simulink library "monroe_library"  (R2012b)
settings: Solver=ode45  StartTime=0.0  StopTime=10.0  RelTol=1e-3
values from neighbouring files (symbols this model uses):
  input_bit_width = ', num2str(input_bit_width))    [fft_direct_draw.m]
undefined symbols (not defined in the file or in its folder): gcbh, xlBlockLoadCallback
libraries: xbsIndex_r4 x1880, monroe_library x159, casper_library x13, xps_library x1
(part 11 of 43)

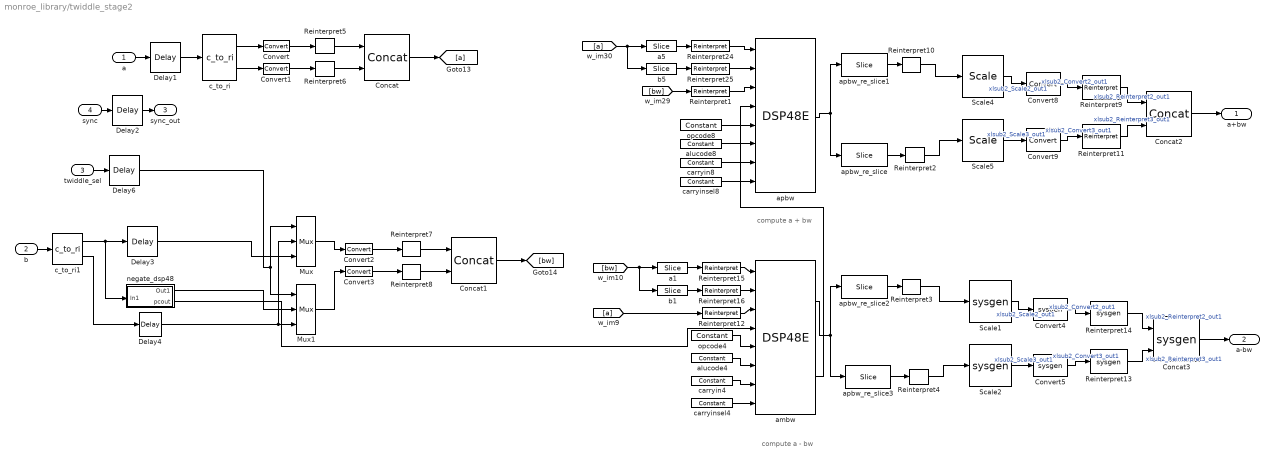
== system monroe_library/twiddle_stage2 ==
  note: compute a + bw
  note: compute a - bw
  a : Inport
  b : Inport  Port=2
  twiddle_sel : Inport  Port=3
  sync : Inport  Port=4
  Concat : xbsIndex_r4/Concat  num_inputs=2  dbl_ovrd=off  block_type=concat
      settings: block_version=11.3
  Concat1 : xbsIndex_r4/Concat  num_inputs=2  dbl_ovrd=off  block_type=concat
      settings: block_version=11.3
  Concat2 : xbsIndex_r4/Concat  num_inputs=2  dbl_ovrd=off  block_type=concat
  Concat3 : S-Function  LoadFcn=xlBlockLoadCallback(gcbh);  FunctionName=sysgen  Parameters=ptable_  EnableBusSupport=off  mask(Xilinx Bus Concatenator Block){infoedit=Concatenates two or more inputs.  Output will be cast to an unsigned value with the binary point at zero., num_inputs=2, dbl_ovrd_sgadvanced=, dbl_ovrd=off, has_advanced_control=0, sggui_pos=-1,-1,-1,-1, block_type=concat, block_version=, sg_icon_stat=60,60,2,1,white,blue,0,16398980,right,,[ ],[ ], sg_mask_display=|, sg_list_contents=, sg_blockgui_xml=}
      mask sg_mask_display=|
      | fprintf('','COMMENT: begin icon graphics');
      | patch([0 60 60 0 0 ],[0 0 60 60 0 ],[0.77 0.82 0.91 ]);
      | plot([0 60 60 0 0 ],[0 0 60 60 0 ]);
      | patch([12.2 23.76 31.76 39.76 47.76 31.76 20.2 12.2 ],[38.88 38.88 46.88 38.88 46.88 46.88 46.88 38.88 ],[1 1 1 ]);
      | patch([20.2 31.76 23.76 12.2 20.2 ],[30.88 30.88 38.88 38.88 30.88 ],[0.931 0.946 0.973 ]);
      | patch([12.2 23.76 31.76 20.2 12.2 ],[22.88 22.88 30.88 30.88 22.88 ],[1 1 1 ]);
      | patch([20.2 47.76 39.76 31.76 23.76 12.2 20.2 ],[14.88 14.88 22.88 14.88 22.88 22.88 14.88 ],[0.931 0.946 0.973 ]);
      | fprintf('','COMMENT: end icon graphics');
      | fprintf('','COMMENT: begin icon text');
      | color('black');port_label('input',1,'hi');
      | color('black');port_label('input',2,'lo');
      |
      | color('black');disp('\fontsize{20}\}','texmode','on');
      | fprintf('','COMMENT: end icon text');
      mask prompts: infoedit ""; num_inputs "Number of inputs"; dbl_ovrd_sgadvanced ""; dbl_ovrd "Override with doubles"; has_advanced_control ""; sggui_pos ""; block_type ""; block_version ""; sg_icon_stat ""; sg_mask_display ""; sg_list_contents ""; sg_blockgui_xml ""
      mask help: Concatenates two or more inputs. Output will be cast to an unsigned value with the binary point at zero.
      mask init: same as monroe_library/double_delay_bram_external_counter/Concat1
      settings: CopyFcn=xlBlockMoveCallback(gcbh);  DeleteFcn=xlDestroyGui(gcbh);  ModelCloseFcn=xlDestroyGui(gcbh);  PreSaveFcn=xlBlockPreSaveCallback(gcbh);  PostSaveFcn=xlBlockPostSaveCallback(gcbh);  DestroyFcn=xlDestroyGui(gcbh);  OpenFcn=xlOpenGui(gcbh, 'concat_gui.xml', @xlmagicenablement, -1)  CloseFcn=xlDestroyGui(gcbh);  MoveFcn=xlBlockMoveCallback(gcbh);
      mask Help: eval('');xlDoc('-book','sysgen','-topic','Concat');
      mask Display:
      | fprintf('','COMMENT: begin icon graphics');
      | patch([0 60 60 0 0 ],[0 0 60 60 0 ],[0.77 0.82 0.91 ]);
      | plot([0 60 60 0 0 ],[0 0 60 60 0 ]);
      | patch([12.2 23.76 31.76 39.76 47.76 31.76 20.2 12.2 ],[38.88 38.88 46.88 38.88 46.88 46.88 46.88 38.88 ],[1 1 1 ]);
      | patch([20.2 31.76 23.76 12.2 20.2 ],[30.88 30.88 38.88 38.88 30.88 ],[0.931 0.946 0.973 ]);
      | patch([12.2 23.76 31.76 20.2 12.2 ],[22.88 22.88 30.88 30.88 22.88 ],[1 1 1 ]);
      | patch([20.2 47.76 39.76 31.76 23.76 12.2 20.2 ],[14.88 14.88 22.88 14.88 22.88 22.88 14.88 ],[0.931 0.946 0.973 ]);
      | fprintf('','COMMENT: end icon graphics');
      | fprintf('','COMMENT: begin icon text');
      | color('black');port_label('input',1,'hi');
      | color('black');port_label('input',2,'lo');
      | 
      | color('black');disp('\fontsize{20}\}','texmode','on');
      | fprintf('','COMMENT: end icon text');
  Convert{,1..3} (4 alike) : xbsIndex_r4/Convert  arith_type="Signed  (2's comp)"  n_bits=24  bin_pt=input_bit_width-1  quantization=Truncate  overflow=Wrap  en=off  latency=0  dbl_ovrd=off  pipeline=off  block_type=convert
      settings: block_version=11.4
  Convert4 : S-Function  LoadFcn=xlBlockLoadCallback(gcbh);  FunctionName=sysgen  Parameters=ptable_  EnableBusSupport=off  mask(Xilinx Type Converter Block){infoedit=Hardware notes: rounding and saturating require hardware resources; truncating and wrapping do not., arith_type_sgadvanced=, arith_type=Signed  (2's comp), n_bits=out_n_bits, bin_pt=out_n_bits-1, quantization_sgadvanced=, quantization=Truncate, overflow_sgadvanced=, overflow=Wrap, en_sgadvanced=, en=off, latency=0, dbl_ovrd_sgadvanced=, dbl_ovrd=off, pipeline_sgadvanced=, pipeline=off, xl_use_area_sgadvanced=, xl_use_area=off, xl_area=[0,0,0,0,0,0,0], has_advanced_control=0, sggui_pos=-1,-1,-1,-1, block_type=convert, block_version=, sg_icon_stat=45,30,1,1,white,blue,0,edca21da,right,,[ ],[ ], sg_mask_display=|, sg_list_contents=, sg_blockgui_xml=}
      mask sg_mask_display=|
      | fprintf('','COMMENT: begin icon graphics');
      | patch([0 45 45 0 0 ],[0 0 30 30 0 ],[0.77 0.82 0.91 ]);
      | plot([0 45 45 0 0 ],[0 0 30 30 0 ]);
      | patch([13.1 18.88 22.88 26.88 30.88 22.88 17.1 13.1 ],[19.44 19.44 23.44 19.44 23.44 23.44 23.44 19.44 ],[1 1 1 ]);
      | patch([17.1 22.88 18.88 13.1 17.1 ],[15.44 15.44 19.44 19.44 15.44 ],[0.931 0.946 0.973 ]);
      | patch([13.1 18.88 22.88 17.1 13.1 ],[11.44 11.44 15.44 15.44 11.44 ],[1 1 1 ]);
      | patch([17.1 30.88 26.88 22.88 18.88 13.1 17.1 ],[7.44 7.44 11.44 7.44 11.44 11.44 7.44 ],[0.931 0.946 0.973 ]);
      | fprintf('','COMMENT: end icon graphics');
      | fprintf('','COMMENT: begin icon text');
      |
      | color('black');port_label('output',1,'cast');
      | fprintf('','COMMENT: end icon text');
      mask prompts: infoedit ""; arith_type_sgadvanced ""; arith_type "Type"; n_bits "Number of bits"; bin_pt "Binary point"; quantization_sgadvanced ""; overflow_sgadvanced ""; en_sgadvanced ""; en "Provide enable port"; dbl_ovrd_sgadvanced ""; dbl_ovrd "Override with doubles"; pipeline_sgadvanced ""; pipeline "Pipeline for maximum performance"; xl_use_area_sgadvanced ""; xl_use_area "Define FPGA area for resource estimation"; xl_area "FPGA area [slices, FFs, BRAMs, LUTs, IOBs, emb. mults, TBUFs]"; has_advanced_control ""; sggui_pos ""; block_type ""; block_version ""; sg_icon_stat ""; sg_mask_display ""; sg_list_contents ""; sg_blockgui_xml ""
      mask help: Hardware notes: rounding and saturating require hardware resources; truncating and wrapping do not.
      mask init: same as monroe_library/dsp48e_mult_add_pcin/Convert
      settings: CopyFcn=xlBlockMoveCallback(gcbh);  DeleteFcn=xlDestroyGui(gcbh);  ModelCloseFcn=xlDestroyGui(gcbh);  PreSaveFcn=xlBlockPreSaveCallback(gcbh);  PostSaveFcn=xlBlockPostSaveCallback(gcbh);  DestroyFcn=xlDestroyGui(gcbh);  OpenFcn=xlOpenGui(gcbh, 'convert_gui.xml', @convertenablement, -1)  CloseFcn=xlDestroyGui(gcbh);  MoveFcn=xlBlockMoveCallback(gcbh);
      mask Help: eval('');xlDoc('-book','sysgen','-topic','Convert');
      mask TypeOptions arith_type: Boolean | Signed  (2's comp) | Unsigned
      mask TypeOptions quantization: Truncate | Round  (unbiased: +/- Inf) | Round  (unbiased: Even Values)
      mask TypeOptions overflow: Wrap | Saturate | Flag as error
      mask Display:
      | fprintf('','COMMENT: begin icon graphics');
      | patch([0 45 45 0 0 ],[0 0 30 30 0 ],[0.77 0.82 0.91 ]);
      | plot([0 45 45 0 0 ],[0 0 30 30 0 ]);
      | patch([13.1 18.88 22.88 26.88 30.88 22.88 17.1 13.1 ],[19.44 19.44 23.44 19.44 23.44 23.44 23.44 19.44 ],[1 1 1 ]);
      | patch([17.1 22.88 18.88 13.1 17.1 ],[15.44 15.44 19.44 19.44 15.44 ],[0.931 0.946 0.973 ]);
      | patch([13.1 18.88 22.88 17.1 13.1 ],[11.44 11.44 15.44 15.44 11.44 ],[1 1 1 ]);
      | patch([17.1 30.88 26.88 22.88 18.88 13.1 17.1 ],[7.44 7.44 11.44 7.44 11.44 11.44 7.44 ],[0.931 0.946 0.973 ]);
      | fprintf('','COMMENT: end icon graphics');
      | fprintf('','COMMENT: begin icon text');
      | 
      | color('black');port_label('output',1,'cast');
      | fprintf('','COMMENT: end icon text');
  Convert5 : S-Function  LoadFcn=xlBlockLoadCallback(gcbh);  FunctionName=sysgen  Parameters=ptable_  EnableBusSupport=off  mask(Xilinx Type Converter Block){infoedit=Hardware notes: rounding and saturating require hardware resources; truncating and wrapping do not., arith_type_sgadvanced=, arith_type=Signed  (2's comp), n_bits=out_n_bits, bin_pt=out_n_bits-1, quantization_sgadvanced=, quantization=Truncate, overflow_sgadvanced=, overflow=Wrap, en_sgadvanced=, en=off, latency=0, dbl_ovrd_sgadvanced=, dbl_ovrd=off, pipeline_sgadvanced=, pipeline=off, xl_use_area_sgadvanced=, xl_use_area=off, xl_area=[0,0,0,0,0,0,0], has_advanced_control=0, sggui_pos=-1,-1,-1,-1, block_type=convert, block_version=, sg_icon_stat=45,30,1,1,white,blue,0,edca21da,right,,[ ],[ ], sg_mask_display=|, sg_list_contents=, sg_blockgui_xml=}
      mask sg_mask_display=|
      | fprintf('','COMMENT: begin icon graphics');
      | patch([0 45 45 0 0 ],[0 0 30 30 0 ],[0.77 0.82 0.91 ]);
      | plot([0 45 45 0 0 ],[0 0 30 30 0 ]);
      | patch([13.1 18.88 22.88 26.88 30.88 22.88 17.1 13.1 ],[19.44 19.44 23.44 19.44 23.44 23.44 23.44 19.44 ],[1 1 1 ]);
      | patch([17.1 22.88 18.88 13.1 17.1 ],[15.44 15.44 19.44 19.44 15.44 ],[0.931 0.946 0.973 ]);
      | patch([13.1 18.88 22.88 17.1 13.1 ],[11.44 11.44 15.44 15.44 11.44 ],[1 1 1 ]);
      | patch([17.1 30.88 26.88 22.88 18.88 13.1 17.1 ],[7.44 7.44 11.44 7.44 11.44 11.44 7.44 ],[0.931 0.946 0.973 ]);
      | fprintf('','COMMENT: end icon graphics');
      | fprintf('','COMMENT: begin icon text');
      |
      | color('black');port_label('output',1,'cast');
      | fprintf('','COMMENT: end icon text');
      mask prompts: infoedit ""; arith_type_sgadvanced ""; arith_type "Type"; n_bits "Number of bits"; bin_pt "Binary point"; quantization_sgadvanced ""; overflow_sgadvanced ""; en_sgadvanced ""; en "Provide enable port"; dbl_ovrd_sgadvanced ""; dbl_ovrd "Override with doubles"; pipeline_sgadvanced ""; pipeline "Pipeline for maximum performance"; xl_use_area_sgadvanced ""; xl_use_area "Define FPGA area for resource estimation"; xl_area "FPGA area [slices, FFs, BRAMs, LUTs, IOBs, emb. mults, TBUFs]"; has_advanced_control ""; sggui_pos ""; block_type ""; block_version ""; sg_icon_stat ""; sg_mask_display ""; sg_list_contents ""; sg_blockgui_xml ""
      mask help: Hardware notes: rounding and saturating require hardware resources; truncating and wrapping do not.
      mask init: same as monroe_library/dsp48e_mult_add_pcin/Convert
      settings: CopyFcn=xlBlockMoveCallback(gcbh);  DeleteFcn=xlDestroyGui(gcbh);  ModelCloseFcn=xlDestroyGui(gcbh);  PreSaveFcn=xlBlockPreSaveCallback(gcbh);  PostSaveFcn=xlBlockPostSaveCallback(gcbh);  DestroyFcn=xlDestroyGui(gcbh);  OpenFcn=xlOpenGui(gcbh, 'convert_gui.xml', @convertenablement, -1)  CloseFcn=xlDestroyGui(gcbh);  MoveFcn=xlBlockMoveCallback(gcbh);
      mask Help: eval('');xlDoc('-book','sysgen','-topic','Convert');
      mask TypeOptions arith_type: Boolean | Signed  (2's comp) | Unsigned
      mask TypeOptions quantization: Truncate | Round  (unbiased: +/- Inf) | Round  (unbiased: Even Values)
      mask TypeOptions overflow: Wrap | Saturate | Flag as error
      mask Display:
      | fprintf('','COMMENT: begin icon graphics');
      | patch([0 45 45 0 0 ],[0 0 30 30 0 ],[0.77 0.82 0.91 ]);
      | plot([0 45 45 0 0 ],[0 0 30 30 0 ]);
      | patch([13.1 18.88 22.88 26.88 30.88 22.88 17.1 13.1 ],[19.44 19.44 23.44 19.44 23.44 23.44 23.44 19.44 ],[1 1 1 ]);
      | patch([17.1 22.88 18.88 13.1 17.1 ],[15.44 15.44 19.44 19.44 15.44 ],[0.931 0.946 0.973 ]);
      | patch([13.1 18.88 22.88 17.1 13.1 ],[11.44 11.44 15.44 15.44 11.44 ],[1 1 1 ]);
      | patch([17.1 30.88 26.88 22.88 18.88 13.1 17.1 ],[7.44 7.44 11.44 7.44 11.44 11.44 7.44 ],[0.931 0.946 0.973 ]);
      | fprintf('','COMMENT: end icon graphics');
      | fprintf('','COMMENT: begin icon text');
      | 
      | color('black');port_label('output',1,'cast');
      | fprintf('','COMMENT: end icon text');
  Convert8 : xbsIndex_r4/Convert  arith_type="Signed  (2's comp)"  n_bits=out_n_bits  bin_pt=out_n_bits-1  quantization=Truncate  overflow=Wrap  en=off  latency=0  dbl_ovrd=off  pipeline=off  block_type=convert
  Convert9 : xbsIndex_r4/Convert  arith_type="Signed  (2's comp)"  n_bits=out_n_bits  bin_pt=out_n_bits-1  quantization=Truncate  overflow=Wrap  en=off  latency=0  dbl_ovrd=off  pipeline=off  block_type=convert
  Delay{1,3..4,6} (4 alike) : xbsIndex_r4/Delay  en=off  latency=3  dbl_ovrd=off  reg_retiming=off  block_type=delay
      settings: xl_area=[0, 0, 0, 0, 0, 0, 0]  block_version=9.1.01
  Delay2 : xbsIndex_r4/Delay  en=off  latency=5  dbl_ovrd=off  reg_retiming=off  block_type=delay
      settings: xl_area=[0, 0, 0, 0, 0, 0, 0]  block_version=9.1.01
  Mux : xbsIndex_r4/Mux  inputs=2  en=off  latency=0  precision=Full  arith_type="Signed  (2's comp)"  n_bits=8  bin_pt=2  quantization=Truncate  overflow=Wrap  dbl_ovrd=off  block_type=mux
      settings: xl_area=[0, 0, 0, 0, 0, 0, 0]  block_version=9.1.01
  Mux1 : xbsIndex_r4/Mux  inputs=2  en=off  latency=0  precision=Full  arith_type="Signed  (2's comp)"  n_bits=8  bin_pt=2  quantization=Truncate  overflow=Wrap  dbl_ovrd=off  block_type=mux
      settings: xl_area=[0, 0, 0, 0, 0, 0, 0]  block_version=9.1.01
  Reinterpret{1,12,15..16,24..25} (6 alike) : xbsIndex_r4/Reinterpret  force_arith_type=on  arith_type="Signed  (2's comp)"  force_bin_pt=off  bin_pt=0  block_type=reinterpret
      settings: infoedit="Changes signal type without altering the binary representation.   You can changed the signal between signed and unsigned, and relocate the binary point.<br><br>Hardware notes: In hardware this block costs nothing.<br><br>Example:  Suppose the input is 6 bits wide, signed, with 2 fractional bits, and the output is forced to unsigned with 0 fractional bits.  Then an input of -2.0 (1110.00 in binary 2's complement) becomes an output of 56 (111000 in binary)."  block_version=11.3
  Reinterpret{2..4,10} (4 alike) : xbsIndex_r4/Reinterpret  force_arith_type=on  arith_type="Signed  (2's comp)"  force_bin_pt=on  bin_pt=input_bit_width-1  block_type=reinterpret
      settings: infoedit="Changes signal type without altering the binary representation.   You can changed the signal between signed and unsigned, and relocate the binary point.<br><br>Hardware notes: In hardware this block costs nothing.<br><br>Example:  Suppose the input is 6 bits wide, signed, with 2 fractional bits, and the output is forced to unsigned with 0 fractional bits.  Then an input of -2.0 (1110.00 in binary 2's complement) becomes an output of 56 (111000 in binary)."  block_version=11.3
  Reinterpret{5..9,11} (6 alike) : xbsIndex_r4/Reinterpret  force_arith_type=on  arith_type=Unsigned  force_bin_pt=on  bin_pt=0  block_type=reinterpret
      Reinterpret11 settings: infoedit="Changes signal type without altering the binary representation.   You can changed the signal between signed and unsigned, and relocate the binary point.<br><br>Hardware notes: In hardware this block costs nothing.<br><br>Example:  Suppose the input is 6 bits wide, signed, with 2 fractional bits, and the output is forced to unsigned with 0 fractional bits.  Then an input of -2.0 (1110.00 in binary 2's complement) becomes an output of 56 (111000 in binary)."
      Reinterpret5 settings: infoedit="Changes signal type without altering the binary representation.   You can changed the signal between signed and unsigned, and relocate the binary point.<br><br>Hardware notes: In hardware this block costs nothing.<br><br>Example:  Suppose the input is 6 bits wide, signed, with 2 fractional bits, and the output is forced to unsigned with 0 fractional bits.  Then an input of -2.0 (1110.00 in binary 2's complement) becomes an output of 56 (111000 in binary)."  block_version=11.3
      Reinterpret6 settings: infoedit="Changes signal type without altering the binary representation.   You can changed the signal between signed and unsigned, and relocate the binary point.<br><br>Hardware notes: In hardware this block costs nothing.<br><br>Example:  Suppose the input is 6 bits wide, signed, with 2 fractional bits, and the output is forced to unsigned with 0 fractional bits.  Then an input of -2.0 (1110.00 in binary 2's complement) becomes an output of 56 (111000 in binary)."  block_version=11.3
      Reinterpret7 settings: infoedit="Changes signal type without altering the binary representation.   You can changed the signal between signed and unsigned, and relocate the binary point.<br><br>Hardware notes: In hardware this block costs nothing.<br><br>Example:  Suppose the input is 6 bits wide, signed, with 2 fractional bits, and the output is forced to unsigned with 0 fractional bits.  Then an input of -2.0 (1110.00 in binary 2's complement) becomes an output of 56 (111000 in binary)."  block_version=11.3
      Reinterpret8 settings: infoedit="Changes signal type without altering the binary representation.   You can changed the signal between signed and unsigned, and relocate the binary point.<br><br>Hardware notes: In hardware this block costs nothing.<br><br>Example:  Suppose the input is 6 bits wide, signed, with 2 fractional bits, and the output is forced to unsigned with 0 fractional bits.  Then an input of -2.0 (1110.00 in binary 2's complement) becomes an output of 56 (111000 in binary)."  block_version=11.3
      Reinterpret9 settings: infoedit="Changes signal type without altering the binary representation.   You can changed the signal between signed and unsigned, and relocate the binary point.<br><br>Hardware notes: In hardware this block costs nothing.<br><br>Example:  Suppose the input is 6 bits wide, signed, with 2 fractional bits, and the output is forced to unsigned with 0 fractional bits.  Then an input of -2.0 (1110.00 in binary 2's complement) becomes an output of 56 (111000 in binary)."
  Reinterpret13 : S-Function  LoadFcn=xlBlockLoadCallback(gcbh);  FunctionName=sysgen  Parameters=ptable_  EnableBusSupport=off  mask(Xilinx Type Reinterpreter Block){infoedit=Changes signal type without altering the binary representation.   You can changed the signal between signed and unsigned, and relocate the binary point.<br><br>Hardware notes: In hardware this block costs nothing.<br><br>Example:  Suppose the input is 6 bits wide, signed, with 2 fractional bits, and the output is forced to unsigned with 0 fractional bits.  Then an input of -2.0 (1110.00 in binary 2's complement) becomes an output of 56 (111000 in binary)., force_arith_type_sgadvanced=, force_arith_type=on, arith_type_sgadvanced=, arith_type=Unsigned, force_bin_pt_sgadvanced=, force_bin_pt=on, bin_pt=0, has_advanced_control=0, sggui_pos=-1,-1,-1,-1, block_type=reinterpret, block_version=, sg_icon_stat=50,32,1,1,white,blue,0,6b04d0b0,right,,[ ],[ ], sg_mask_display=|, sg_list_contents=, sg_blockgui_xml=}
      mask sg_mask_display=|
      | fprintf('','COMMENT: begin icon graphics');
      | patch([0 50 50 0 0 ],[0 0 32 32 0 ],[0.77 0.82 0.91 ]);
      | plot([0 50 50 0 0 ],[0 0 32 32 0 ]);
      | patch([16.1 21.88 25.88 29.88 33.88 25.88 20.1 16.1 ],[20.44 20.44 24.44 20.44 24.44 24.44 24.44 20.44 ],[1 1 1 ]);
      | patch([20.1 25.88 21.88 16.1 20.1 ],[16.44 16.44 20.44 20.44 16.44 ],[0.931 0.946 0.973 ]);
      | patch([16.1 21.88 25.88 20.1 16.1 ],[12.44 12.44 16.44 16.44 12.44 ],[1 1 1 ]);
      | patch([20.1 33.88 29.88 25.88 21.88 16.1 20.1 ],[8.44 8.44 12.44 8.44 12.44 12.44 8.44 ],[0.931 0.946 0.973 ]);
      | fprintf('','COMMENT: end icon graphics');
      | fprintf('','COMMENT: begin icon text');
      |
      |
      | color('black');disp('reinterpret');
      | fprintf('','COMMENT: end icon text');
      mask prompts: infoedit ""; force_arith_type_sgadvanced ""; force_arith_type "Force Arithmetic Type"; arith_type_sgadvanced ""; arith_type "Output Arithmetic Type"; force_bin_pt_sgadvanced ""; force_bin_pt "Force Binary Point"; bin_pt "Output Binary Point"; has_advanced_control ""; sggui_pos ""; block_type ""; block_version ""; sg_icon_stat ""; sg_mask_display ""; sg_list_contents ""; sg_blockgui_xml ""
      mask help:
      | Changes signal type without altering the binary representation.   You can changed the signal between signed and unsigned, and relocate the binary point.
      |
      | Hardware notes: In hardware this block costs nothing.
      |
      | Example:  Suppose the input is 6 bits wide, signed, with 2 fractional bits, and the output is forced to unsigned with 0 fractional bits.  Then an input of -2.0 (1110.00 in binary 2's complement) becomes an output of 56 (111000 in binary).
      mask init: same as monroe_library/twiddle_cheap/Reinterpret4
      settings: CopyFcn=xlBlockMoveCallback(gcbh);  DeleteFcn=xlDestroyGui(gcbh);  ModelCloseFcn=xlDestroyGui(gcbh);  PreSaveFcn=xlBlockPreSaveCallback(gcbh);  PostSaveFcn=xlBlockPostSaveCallback(gcbh);  DestroyFcn=xlDestroyGui(gcbh);  OpenFcn=xlOpenGui(gcbh, 'reinterpret_gui.xml', @reinterpretenablement, -1)  CloseFcn=xlDestroyGui(gcbh);  MoveFcn=xlBlockMoveCallback(gcbh);
      mask Help: eval('');xlDoc('-book','sysgen','-topic','Reinterpret');
      mask TypeOptions arith_type: Unsigned | Signed  (2's comp)
      mask Display:
      | fprintf('','COMMENT: begin icon graphics');
      | patch([0 50 50 0 0 ],[0 0 32 32 0 ],[0.77 0.82 0.91 ]);
      | plot([0 50 50 0 0 ],[0 0 32 32 0 ]);
      | patch([16.1 21.88 25.88 29.88 33.88 25.88 20.1 16.1 ],[20.44 20.44 24.44 20.44 24.44 24.44 24.44 20.44 ],[1 1 1 ]);
      | patch([20.1 25.88 21.88 16.1 20.1 ],[16.44 16.44 20.44 20.44 16.44 ],[0.931 0.946 0.973 ]);
      | patch([16.1 21.88 25.88 20.1 16.1 ],[12.44 12.44 16.44 16.44 12.44 ],[1 1 1 ]);
      | patch([20.1 33.88 29.88 25.88 21.88 16.1 20.1 ],[8.44 8.44 12.44 8.44 12.44 12.44 8.44 ],[0.931 0.946 0.973 ]);
      | fprintf('','COMMENT: end icon graphics');
      | fprintf('','COMMENT: begin icon text');
      | 
      | 
      | color('black');disp('reinterpret');
      | fprintf('','COMMENT: end icon text');
  Reinterpret14 : S-Function  LoadFcn=xlBlockLoadCallback(gcbh);  FunctionName=sysgen  Parameters=ptable_  EnableBusSupport=off  mask(Xilinx Type Reinterpreter Block){infoedit=Changes signal type without altering the binary representation.   You can changed the signal between signed and unsigned, and relocate the binary point.<br><br>Hardware notes: In hardware this block costs nothing.<br><br>Example:  Suppose the input is 6 bits wide, signed, with 2 fractional bits, and the output is forced to unsigned with 0 fractional bits.  Then an input of -2.0 (1110.00 in binary 2's complement) becomes an output of 56 (111000 in binary)., force_arith_type_sgadvanced=, force_arith_type=on, arith_type_sgadvanced=, arith_type=Unsigned, force_bin_pt_sgadvanced=, force_bin_pt=on, bin_pt=0, has_advanced_control=0, sggui_pos=-1,-1,-1,-1, block_type=reinterpret, block_version=, sg_icon_stat=50,32,1,1,white,blue,0,6b04d0b0,right,,[ ],[ ], sg_mask_display=|, sg_list_contents=, sg_blockgui_xml=}
      mask sg_mask_display=|
      | fprintf('','COMMENT: begin icon graphics');
      | patch([0 50 50 0 0 ],[0 0 32 32 0 ],[0.77 0.82 0.91 ]);
      | plot([0 50 50 0 0 ],[0 0 32 32 0 ]);
      | patch([16.1 21.88 25.88 29.88 33.88 25.88 20.1 16.1 ],[20.44 20.44 24.44 20.44 24.44 24.44 24.44 20.44 ],[1 1 1 ]);
      | patch([20.1 25.88 21.88 16.1 20.1 ],[16.44 16.44 20.44 20.44 16.44 ],[0.931 0.946 0.973 ]);
      | patch([16.1 21.88 25.88 20.1 16.1 ],[12.44 12.44 16.44 16.44 12.44 ],[1 1 1 ]);
      | patch([20.1 33.88 29.88 25.88 21.88 16.1 20.1 ],[8.44 8.44 12.44 8.44 12.44 12.44 8.44 ],[0.931 0.946 0.973 ]);
      | fprintf('','COMMENT: end icon graphics');
      | fprintf('','COMMENT: begin icon text');
      |
      |
      | color('black');disp('reinterpret');
      | fprintf('','COMMENT: end icon text');
      mask prompts: infoedit ""; force_arith_type_sgadvanced ""; force_arith_type "Force Arithmetic Type"; arith_type_sgadvanced ""; arith_type "Output Arithmetic Type"; force_bin_pt_sgadvanced ""; force_bin_pt "Force Binary Point"; bin_pt "Output Binary Point"; has_advanced_control ""; sggui_pos ""; block_type ""; block_version ""; sg_icon_stat ""; sg_mask_display ""; sg_list_contents ""; sg_blockgui_xml ""
      mask help:
      | Changes signal type without altering the binary representation.   You can changed the signal between signed and unsigned, and relocate the binary point.
      |
      | Hardware notes: In hardware this block costs nothing.
      |
      | Example:  Suppose the input is 6 bits wide, signed, with 2 fractional bits, and the output is forced to unsigned with 0 fractional bits.  Then an input of -2.0 (1110.00 in binary 2's complement) becomes an output of 56 (111000 in binary).
      mask init: same as monroe_library/twiddle_cheap/Reinterpret4
      settings: CopyFcn=xlBlockMoveCallback(gcbh);  DeleteFcn=xlDestroyGui(gcbh);  ModelCloseFcn=xlDestroyGui(gcbh);  PreSaveFcn=xlBlockPreSaveCallback(gcbh);  PostSaveFcn=xlBlockPostSaveCallback(gcbh);  DestroyFcn=xlDestroyGui(gcbh);  OpenFcn=xlOpenGui(gcbh, 'reinterpret_gui.xml', @reinterpretenablement, -1)  CloseFcn=xlDestroyGui(gcbh);  MoveFcn=xlBlockMoveCallback(gcbh);
      mask Help: eval('');xlDoc('-book','sysgen','-topic','Reinterpret');
      mask TypeOptions arith_type: Unsigned | Signed  (2's comp)
      mask Display:
      | fprintf('','COMMENT: begin icon graphics');
      | patch([0 50 50 0 0 ],[0 0 32 32 0 ],[0.77 0.82 0.91 ]);
      | plot([0 50 50 0 0 ],[0 0 32 32 0 ]);
      | patch([16.1 21.88 25.88 29.88 33.88 25.88 20.1 16.1 ],[20.44 20.44 24.44 20.44 24.44 24.44 24.44 20.44 ],[1 1 1 ]);
      | patch([20.1 25.88 21.88 16.1 20.1 ],[16.44 16.44 20.44 20.44 16.44 ],[0.931 0.946 0.973 ]);
      | patch([16.1 21.88 25.88 20.1 16.1 ],[12.44 12.44 16.44 16.44 12.44 ],[1 1 1 ]);
      | patch([20.1 33.88 29.88 25.88 21.88 16.1 20.1 ],[8.44 8.44 12.44 8.44 12.44 12.44 8.44 ],[0.931 0.946 0.973 ]);
      | fprintf('','COMMENT: end icon graphics');
      | fprintf('','COMMENT: begin icon text');
      | 
      | 
      | color('black');disp('reinterpret');
      | fprintf('','COMMENT: end icon text');
  Scale1 : S-Function  LoadFcn=xlBlockLoadCallback(gcbh);  FunctionName=sysgen  Parameters=ptable_  EnableBusSupport=off  mask(Xilinx Input Scaler Block){infoedit=Scales input by a power of two by adjusting the binary point position.<br><br>Hardware notes: In hardware this block costs nothing., scale_factor=downshift_at_end*-1, dbl_ovrd_sgadvanced=, dbl_ovrd=off, has_advanced_control=0, sggui_pos=-1,-1,-1,-1, block_type=scale, block_version=, sg_icon_stat=55,56,1,1,white,blue,0,e7f93c29,right,,[ ],[ ], sg_mask_display=|, sg_list_contents=, sg_blockgui_xml=}
      mask sg_mask_display=|
      | fprintf('','COMMENT: begin icon graphics');
      | patch([0 55 55 0 0 ],[0 0 56 56 0 ],[0.77 0.82 0.91 ]);
      | plot([0 55 55 0 0 ],[0 0 56 56 0 ]);
      | patch([11.425 21.54 28.54 35.54 42.54 28.54 18.425 11.425 ],[35.77 35.77 42.77 35.77 42.77 42.77 42.77 35.77 ],[1 1 1 ]);
      | patch([18.425 28.54 21.54 11.425 18.425 ],[28.77 28.77 35.77 35.77 28.77 ],[0.931 0.946 0.973 ]);
      | patch([11.425 21.54 28.54 18.425 11.425 ],[21.77 21.77 28.77 28.77 21.77 ],[1 1 1 ]);
      | patch([18.425 42.54 35.54 28.54 21.54 11.425 18.425 ],[14.77 14.77 21.77 14.77 21.77 21.77 14.77 ],[0.931 0.946 0.973 ]);
      | fprintf('','COMMENT: end icon graphics');
      | fprintf('','COMMENT: begin icon text');
      |
      |
      | color('black');disp('\bf{2^{0}}','texmode','on');
      | fprintf('','COMMENT: end icon text');
      mask prompts: infoedit ""; scale_factor "Scale factor s (scale output by 2^s)"; dbl_ovrd_sgadvanced ""; dbl_ovrd "Override with doubles"; has_advanced_control ""; sggui_pos ""; block_type ""; block_version ""; sg_icon_stat ""; sg_mask_display ""; sg_list_contents ""; sg_blockgui_xml ""
      mask help:
      | Scales input by a power of two by adjusting the binary point position.
      |
      | Hardware notes: In hardware this block costs nothing.
      mask init: same as monroe_library/twiddle_cheap/Scale6
      settings: CopyFcn=xlBlockMoveCallback(gcbh);  DeleteFcn=xlDestroyGui(gcbh);  ModelCloseFcn=xlDestroyGui(gcbh);  PreSaveFcn=xlBlockPreSaveCallback(gcbh);  PostSaveFcn=xlBlockPostSaveCallback(gcbh);  DestroyFcn=xlDestroyGui(gcbh);  OpenFcn=xlOpenGui(gcbh, 'scale_gui.xml', @xlmagicenablement, -1)  CloseFcn=xlDestroyGui(gcbh);  MoveFcn=xlBlockMoveCallback(gcbh);
      mask Help: eval('');xlDoc('-book','sysgen','-topic','Scale');
      mask Display:
      | fprintf('','COMMENT: begin icon graphics');
      | patch([0 55 55 0 0 ],[0 0 56 56 0 ],[0.77 0.82 0.91 ]);
      | plot([0 55 55 0 0 ],[0 0 56 56 0 ]);
      | patch([11.425 21.54 28.54 35.54 42.54 28.54 18.425 11.425 ],[35.77 35.77 42.77 35.77 42.77 42.77 42.77 35.77 ],[1 1 1 ]);
      | patch([18.425 28.54 21.54 11.425 18.425 ],[28.77 28.77 35.77 35.77 28.77 ],[0.931 0.946 0.973 ]);
      | patch([11.425 21.54 28.54 18.425 11.425 ],[21.77 21.77 28.77 28.77 21.77 ],[1 1 1 ]);
      | patch([18.425 42.54 35.54 28.54 21.54 11.425 18.425 ],[14.77 14.77 21.77 14.77 21.77 21.77 14.77 ],[0.931 0.946 0.973 ]);
      | fprintf('','COMMENT: end icon graphics');
      | fprintf('','COMMENT: begin icon text');
      | 
      | 
      | color('black');disp('\bf{2^{0}}','texmode','on');
      | fprintf('','COMMENT: end icon text');
  Scale2 : S-Function  LoadFcn=xlBlockLoadCallback(gcbh);  FunctionName=sysgen  Parameters=ptable_  EnableBusSupport=off  mask(Xilinx Input Scaler Block){infoedit=Scales input by a power of two by adjusting the binary point position.<br><br>Hardware notes: In hardware this block costs nothing., scale_factor=downshift_at_end*-1, dbl_ovrd_sgadvanced=, dbl_ovrd=off, has_advanced_control=0, sggui_pos=-1,-1,-1,-1, block_type=scale, block_version=, sg_icon_stat=55,56,1,1,white,blue,0,e7f93c29,right,,[ ],[ ], sg_mask_display=|, sg_list_contents=, sg_blockgui_xml=}
      mask sg_mask_display=|
      | fprintf('','COMMENT: begin icon graphics');
      | patch([0 55 55 0 0 ],[0 0 56 56 0 ],[0.77 0.82 0.91 ]);
      | plot([0 55 55 0 0 ],[0 0 56 56 0 ]);
      | patch([11.425 21.54 28.54 35.54 42.54 28.54 18.425 11.425 ],[35.77 35.77 42.77 35.77 42.77 42.77 42.77 35.77 ],[1 1 1 ]);
      | patch([18.425 28.54 21.54 11.425 18.425 ],[28.77 28.77 35.77 35.77 28.77 ],[0.931 0.946 0.973 ]);
      | patch([11.425 21.54 28.54 18.425 11.425 ],[21.77 21.77 28.77 28.77 21.77 ],[1 1 1 ]);
      | patch([18.425 42.54 35.54 28.54 21.54 11.425 18.425 ],[14.77 14.77 21.77 14.77 21.77 21.77 14.77 ],[0.931 0.946 0.973 ]);
      | fprintf('','COMMENT: end icon graphics');
      | fprintf('','COMMENT: begin icon text');
      |
      |
      | color('black');disp('\bf{2^{0}}','texmode','on');
      | fprintf('','COMMENT: end icon text');
      mask prompts: infoedit ""; scale_factor "Scale factor s (scale output by 2^s)"; dbl_ovrd_sgadvanced ""; dbl_ovrd "Override with doubles"; has_advanced_control ""; sggui_pos ""; block_type ""; block_version ""; sg_icon_stat ""; sg_mask_display ""; sg_list_contents ""; sg_blockgui_xml ""
      mask help:
      | Scales input by a power of two by adjusting the binary point position.
      |
      | Hardware notes: In hardware this block costs nothing.
      mask init: same as monroe_library/twiddle_cheap/Scale6
      settings: CopyFcn=xlBlockMoveCallback(gcbh);  DeleteFcn=xlDestroyGui(gcbh);  ModelCloseFcn=xlDestroyGui(gcbh);  PreSaveFcn=xlBlockPreSaveCallback(gcbh);  PostSaveFcn=xlBlockPostSaveCallback(gcbh);  DestroyFcn=xlDestroyGui(gcbh);  OpenFcn=xlOpenGui(gcbh, 'scale_gui.xml', @xlmagicenablement, -1)  CloseFcn=xlDestroyGui(gcbh);  MoveFcn=xlBlockMoveCallback(gcbh);
      mask Help: eval('');xlDoc('-book','sysgen','-topic','Scale');
      mask Display:
      | fprintf('','COMMENT: begin icon graphics');
      | patch([0 55 55 0 0 ],[0 0 56 56 0 ],[0.77 0.82 0.91 ]);
      | plot([0 55 55 0 0 ],[0 0 56 56 0 ]);
      | patch([11.425 21.54 28.54 35.54 42.54 28.54 18.425 11.425 ],[35.77 35.77 42.77 35.77 42.77 42.77 42.77 35.77 ],[1 1 1 ]);
      | patch([18.425 28.54 21.54 11.425 18.425 ],[28.77 28.77 35.77 35.77 28.77 ],[0.931 0.946 0.973 ]);
      | patch([11.425 21.54 28.54 18.425 11.425 ],[21.77 21.77 28.77 28.77 21.77 ],[1 1 1 ]);
      | patch([18.425 42.54 35.54 28.54 21.54 11.425 18.425 ],[14.77 14.77 21.77 14.77 21.77 21.77 14.77 ],[0.931 0.946 0.973 ]);
      | fprintf('','COMMENT: end icon graphics');
      | fprintf('','COMMENT: begin icon text');
      | 
      | 
      | color('black');disp('\bf{2^{0}}','texmode','on');
      | fprintf('','COMMENT: end icon text');
  Scale4 : xbsIndex_r4/Scale  scale_factor=downshift_at_end*-1  dbl_ovrd=off  block_type=scale
  Scale5 : xbsIndex_r4/Scale  scale_factor=downshift_at_end*-1  dbl_ovrd=off  block_type=scale
  a1 : xbsIndex_r4/Slice  nbits=30  boolean_output=off  mode=Upper Bit Location + Width  bit1=0  base1=MSB of Input  bit0=18  base0=LSB of Input  dbl_ovrd=off  block_type=slice
      settings: block_version=11.3
  a5 : xbsIndex_r4/Slice  nbits=30  boolean_output=off  mode=Upper Bit Location + Width  bit1=0  base1=MSB of Input  bit0=18  base0=LSB of Input  dbl_ovrd=off  block_type=slice
      settings: block_version=11.3
  alucode4 : xbsIndex_r4/Constant  arith_type=Unsigned  const=3  n_bits=4  bin_pt=0  explicit_period=on  period=1  equ=P=C  opselect=C  inp2=PCIN>>17  opr=+  inp1=P  carry=CIN  dbl_ovrd=off  block_type=constant
  alucode8 : xbsIndex_r4/Constant  arith_type=Unsigned  const=0  n_bits=4  bin_pt=0  explicit_period=on  period=1  equ=P=C  opselect=C  inp2=PCIN>>17  opr=+  inp1=P  carry=CIN  dbl_ovrd=off  block_type=constant
  ambw : xbsIndex_r4/DSP48E  use_a=Direct from A Port  use_b=Direct from B Port  reset_preg=off  pattern_from_creg=off  pattern='000000000000'  mask_from_creg=off  pattern_mask='3FFFFFFFFFFF'  sel_rounding_mask=Select mask  use_op=off  use_creg=on  rst_all=off  en_all=off  use_pcin=on  use_carrycascin=off  use_multsignin=off  use_carryout=off  use_patterndetect=off  use_patternbdetect=off  use_overflow=off  use_underflow=off  use_acout=off  use_bcout=off  use_pcout=on  use_multsignout=off  use_carrycascout=off  pipeline_a=1  pipeline_b=1  pipeline_acout=1  pipeline_bcout=1  pipeline_c=on  pipeline_p=on  pipeline_mult=on  pipeline_opmode=on  pipeline_alumode=on  pipeline_carryin=on  pipeline_carryinsel=on  rst_a=off  rst_b=off  rst_c=off  rst_mult=off  rst_p=off  rst_carry_in=off  rst_alumode=off  rst_ctrl=off  en_a1=off  en_a2=off  en_b1=off  en_b2=off  en_c=off  en_mult=off  en_p=off  en_carry_in=off  en_alumode=off  en_multcarryin=off  en_ctrl=off  use_synth_model=off  addsub_mode=TWO24  xl_useadderonly=off  block_type=dsp48e
      settings: block_version=10.1.3
  apbw : xbsIndex_r4/DSP48E  use_a=Direct from A Port  use_b=Direct from B Port  reset_preg=off  pattern_from_creg=off  pattern='000000000000'  mask_from_creg=off  pattern_mask='3FFFFFFFFFFF'  sel_rounding_mask=Select mask  use_op=off  use_creg=on  rst_all=off  en_all=off  use_pcin=on  use_carrycascin=off  use_multsignin=off  use_carryout=off  use_patterndetect=off  use_patternbdetect=off  use_overflow=off  use_underflow=off  use_acout=off  use_bcout=off  use_pcout=off  use_multsignout=off  use_carrycascout=off  pipeline_a=1  pipeline_b=1  pipeline_acout=1  pipeline_bcout=1  pipeline_c=on  pipeline_p=on  pipeline_mult=on  pipeline_opmode=on  pipeline_alumode=on  pipeline_carryin=on  pipeline_carryinsel=on  rst_a=off  rst_b=off  rst_c=off  rst_mult=off  rst_p=off  rst_carry_in=off  rst_alumode=off  rst_ctrl=off  en_a1=off  en_a2=off  en_b1=off  en_b2=off  en_c=off  en_mult=off  en_p=off  en_carry_in=off  en_alumode=off  en_multcarryin=off  en_ctrl=off  use_synth_model=off  addsub_mode=TWO24  xl_useadderonly=off  block_type=dsp48e
      settings: block_version=10.1.3
  apbw_re_slice : xbsIndex_r4/Slice  nbits=24  boolean_output=off  mode=Lower Bit Location + Width  bit1=0  base1=MSB of Input  bit0=0  base0=LSB of Input  dbl_ovrd=off  block_type=slice
      settings: block_version=11.3
  apbw_re_slice1 : xbsIndex_r4/Slice  nbits=24  boolean_output=off  mode=Upper Bit Location + Width  bit1=0  base1=MSB of Input  bit0=24  base0=LSB of Input  dbl_ovrd=off  block_type=slice
      settings: block_version=11.3
  apbw_re_slice2 : xbsIndex_r4/Slice  nbits=24  boolean_output=off  mode=Upper Bit Location + Width  bit1=0  base1=MSB of Input  bit0=24  base0=LSB of Input  dbl_ovrd=off  block_type=slice
      settings: block_version=11.3
  apbw_re_slice3 : xbsIndex_r4/Slice  nbits=24  boolean_output=off  mode=Lower Bit Location + Width  bit1=0  base1=MSB of Input  bit0=0  base0=LSB of Input  dbl_ovrd=off  block_type=slice
      settings: block_version=11.3
  b1 : xbsIndex_r4/Slice  nbits=18  boolean_output=off  mode=Lower Bit Location + Width  bit1=0  base1=MSB of Input  bit0=0  base0=LSB of Input  dbl_ovrd=off  block_type=slice
      settings: block_version=11.3
  b5 : xbsIndex_r4/Slice  nbits=18  boolean_output=off  mode=Lower Bit Location + Width  bit1=0  base1=MSB of Input  bit0=0  base0=LSB of Input  dbl_ovrd=off  block_type=slice
      settings: block_version=11.3
  c_to_ri : casper_library/Misc/c_to_ri  SystemSampleTime=-1  n_bits=input_bit_width  bin_pt=input_bit_width-1
      settings: AttributesFormatString=18_17 r/i
  c_to_ri1 : casper_library/Misc/c_to_ri  SystemSampleTime=-1  n_bits=input_bit_width  bin_pt=input_bit_width-1
      settings: AttributesFormatString=18_17 r/i
  carryin4 : xbsIndex_r4/Constant  arith_type=Unsigned  const=0  n_bits=1  bin_pt=0  explicit_period=on  period=1  equ=P=C  opselect=C  inp2=PCIN>>17  opr=+  inp1=P  carry=CIN  dbl_ovrd=off  block_type=constant
  carryin8 : xbsIndex_r4/Constant  arith_type=Unsigned  const=0  n_bits=1  bin_pt=0  explicit_period=on  period=1  equ=P=C  opselect=C  inp2=PCIN>>17  opr=+  inp1=P  carry=CIN  dbl_ovrd=off  block_type=constant
  carryinsel4 : xbsIndex_r4/Constant  arith_type=Unsigned  const=0  n_bits=3  bin_pt=0  explicit_period=on  period=1  equ=P=C  opselect=C  inp2=PCIN>>17  opr=+  inp1=P  carry=CIN  dbl_ovrd=off  block_type=constant
  carryinsel8 : xbsIndex_r4/Constant  arith_type=Unsigned  const=0  n_bits=3  bin_pt=0  explicit_period=on  period=1  equ=P=C  opselect=C  inp2=PCIN>>17  opr=+  inp1=P  carry=CIN  dbl_ovrd=off  block_type=constant
  negate_dsp48 : Subsystem  mask{input_bit_width=input_bit_width, input_bin_pt=input_bit_width-1}
      mask prompts: input_bit_width "Bit Width"; input_bin_pt "Binary Point"
  opcode4 : xbsIndex_r4/Constant  arith_type=Unsigned  const=51  n_bits=7  bin_pt=0  explicit_period=on  period=1  equ=P=C  opselect=C  inp2=PCIN>>17  opr=+  inp1=P  carry=CIN  dbl_ovrd=off  block_type=constant
  opcode8 : xbsIndex_r4/Constant  arith_type=Unsigned  const=15  n_bits=7  bin_pt=0  explicit_period=on  period=1  equ=P=C  opselect=C  inp2=PCIN>>17  opr=+  inp1=P  carry=CIN  dbl_ovrd=off  block_type=constant
  a+bw : Outport
  a-bw : Outport  Port=2
  sync_out : Outport  Port=3
  wires:
  Delay4/1 -> Mux/2, Mux1/3
  Delay2/1 -> sync_out/1
  Mux1/1 -> Convert3/1
  Mux/1 -> Convert2/1
  c_to_ri1/1 -> negate_dsp48/1(In1), Delay3/1
  Delay6/1 -> Mux/1, Mux1/1
  negate_dsp48/1(Out1) -> Mux1/2
  c_to_ri1/2 -> Delay4/1
  c_to_ri/2 -> Convert1/1
  c_to_ri/1 -> Convert/1
  Delay1/1 -> c_to_ri/1
  b/1 -> c_to_ri1/1
  sync/1 -> Delay2/1
  a/1 -> Delay1/1
  Convert/1 -> Reinterpret5/1
  Convert1/1 -> Reinterpret6/1
  Convert2/1 -> Reinterpret7/1
  Convert3/1 -> Reinterpret8/1
  Reinterpret5/1 -> Concat/1
  Reinterpret6/1 -> Concat/2
  Reinterpret7/1 -> Concat1/1
  Reinterpret8/1 -> Concat1/2
  Concat/1 -> [a]
  Concat1/1 -> [bw]
  apbw_re_slice1/1 -> Reinterpret10/1
  [a] -> b5/1, a5/1
  [bw] -> Reinterpret1/1
  a5/1 -> Reinterpret24/1
  Reinterpret24/1 -> apbw/1
  b5/1 -> Reinterpret25/1
  Reinterpret25/1 -> apbw/2
  apbw/1 -> apbw_re_slice1/1, apbw_re_slice/1
  apbw_re_slice/1 -> Reinterpret2/1
  Reinterpret1/1 -> apbw/3
  apbw_re_slice2/1 -> Reinterpret3/1
  [bw] -> a1/1, b1/1
  [a] -> Reinterpret12/1
  a1/1 -> Reinterpret15/1
  Reinterpret15/1 -> ambw/1
  b1/1 -> Reinterpret16/1
  Reinterpret16/1 -> ambw/2
  ambw/1 -> apbw_re_slice2/1, apbw_re_slice3/1
  apbw_re_slice3/1 -> Reinterpret4/1
  Reinterpret12/1 -> ambw/3
  twiddle_sel/1 -> Delay6/1
  Delay3/1 -> Mux/3
  opcode4/1 -> ambw/5
  alucode4/1 -> ambw/6
  carryin4/1 -> ambw/7
  carryinsel4/1 -> ambw/8
  opcode8/1 -> apbw/5
  alucode8/1 -> apbw/6
  carryin8/1 -> apbw/7
  carryinsel8/1 -> apbw/8
  ambw/2 -> apbw/4
  negate_dsp48/2(pcout) -> ambw/4
  Scale5/1 -> Convert9/1  "xlsub2_Scale3_out1"
  Scale4/1 -> Convert8/1  "xlsub2_Scale2_out1"
  Reinterpret11/1 -> Concat2/2  "xlsub2_Reinterpret3_out1"
  Convert9/1 -> Reinterpret11/1  "xlsub2_Convert3_out1"
  Reinterpret9/1 -> Concat2/1  "xlsub2_Reinterpret2_out1"
  Convert8/1 -> Reinterpret9/1  "xlsub2_Convert2_out1"
  Scale2/1 -> Convert5/1  "xlsub2_Scale3_out1"
  Scale1/1 -> Convert4/1  "xlsub2_Scale2_out1"
  Reinterpret13/1 -> Concat3/2  "xlsub2_Reinterpret3_out1"
  Convert5/1 -> Reinterpret13/1  "xlsub2_Convert3_out1"
  Reinterpret14/1 -> Concat3/1  "xlsub2_Reinterpret2_out1"
  Convert4/1 -> Reinterpret14/1  "xlsub2_Convert2_out1"
  Concat3/1 -> a-bw/1
  Concat2/1 -> a+bw/1
  Reinterpret10/1 -> Scale4/1
  Reinterpret2/1 -> Scale5/1
  Reinterpret3/1 -> Scale1/1
  Reinterpret4/1 -> Scale2/1

== system monroe_library/uncram ==
  in : Inport
  reinterpret1 : xbsIndex_r4/Reinterpret  force_arith_type=on  arith_type="Signed  (2's comp)"  force_bin_pt=on  bin_pt=17  block_type=reinterpret
      settings: infoedit="Changes signal type without altering the binary representation.   You can changed the signal between signed and unsigned, and relocate the binary point.<br><br>Hardware notes: In hardware this block costs nothing.<br><br>Example:  Suppose the input is 6 bits wide, signed, with 2 fractional bits, and the output is forced to unsigned with 0 fractional bits.  Then an input of -2.0 (1110.00 in binary 2's complement) becomes an output of 56 (111000 in binary)."
  reinterpret2 : xbsIndex_r4/Reinterpret  force_arith_type=on  arith_type="Signed  (2's comp)"  force_bin_pt=on  bin_pt=17  block_type=reinterpret
      settings: infoedit="Changes signal type without altering the binary representation.   You can changed the signal between signed and unsigned, and relocate the binary point.<br><br>Hardware notes: In hardware this block costs nothing.<br><br>Example:  Suppose the input is 6 bits wide, signed, with 2 fractional bits, and the output is forced to unsigned with 0 fractional bits.  Then an input of -2.0 (1110.00 in binary 2's complement) becomes an output of 56 (111000 in binary)."
  reinterpret3 : xbsIndex_r4/Reinterpret  force_arith_type=on  arith_type="Signed  (2's comp)"  force_bin_pt=on  bin_pt=17  block_type=reinterpret
      settings: infoedit="Changes signal type without altering the binary representation.   You can changed the signal between signed and unsigned, and relocate the binary point.<br><br>Hardware notes: In hardware this block costs nothing.<br><br>Example:  Suppose the input is 6 bits wide, signed, with 2 fractional bits, and the output is forced to unsigned with 0 fractional bits.  Then an input of -2.0 (1110.00 in binary 2's complement) becomes an output of 56 (111000 in binary)."
  signal1 : xbsIndex_r4/Slice  nbits=18  boolean_output=off  mode=Upper Bit Location + Width  bit1=-0  base1=MSB of Input  bit0=-0  base0=MSB of Input  dbl_ovrd=off  block_type=slice
  signal2 : xbsIndex_r4/Slice  nbits=18  boolean_output=off  mode=Upper Bit Location + Width  bit1=-18  base1=MSB of Input  bit0=-18  base0=MSB of Input  dbl_ovrd=off  block_type=slice
  signal3 : xbsIndex_r4/Slice  nbits=18  boolean_output=off  mode=Upper Bit Location + Width  bit1=-36  base1=MSB of Input  bit0=-36  base0=MSB of Input  dbl_ovrd=off  block_type=slice
  out0 : Outport
  out1 : Outport  Port=2
  out2 : Outport  Port=3
  wires:
  in/1 -> signal3/1, signal2/1, signal1/1
  reinterpret3/1 -> out2/1
  signal3/1 -> reinterpret3/1
  reinterpret2/1 -> out1/1
  signal2/1 -> reinterpret2/1
  reinterpret1/1 -> out0/1
  signal1/1 -> reinterpret1/1

== system monroe_library/unscr_tail ==
  sync : Inport
  In1 : Inport  Port=2
  In2 : Inport  Port=3
  In3 : Inport  Port=4
  In4 : Inport  Port=5
  Delay1 : xbsIndex_r4/Delay  en=off  latency=bram_latency + reorder_din_latency  dbl_ovrd=off  reg_retiming=off  block_type=delay
  complex_addsub1 : Subsystem  mask(complex_addsub){BitWidth=input_bit_width, add_latency=0}
      mask prompts: BitWidth "Bit Wdith"; add_latency "Add Latency"
      mask help:
      | Adds and subtracts the complex inputs.
      | If a = w + ix, b = y + iz then
      | a+b = (w+y)/2 + i(x-z)/2 and
      | a-b = (x+z)/2 + i(y-w)/2
  complex_addsub2 : Subsystem  mask(complex_addsub){BitWidth=input_bit_width, add_latency=0}
      mask prompts: BitWidth "Bit Wdith"; add_latency "Add Latency"
      mask help:
      | Adds and subtracts the complex inputs.
      | If a = w + ix, b = y + iz then
      | a+b = (w+y)/2 + i(x-z)/2 and
      | a-b = (x+z)/2 + i(y-w)/2
  mirror_spectrum : Subsystem
  reorder2 : Subsystem
  sync_delay_fast : monroe_library/sync_delay_fast  SystemSampleTime=-1  delay_len=2^(FFTSize-1)
  sync_out : Outport
  pol1_out : Outport  Port=2
  pol2_out : Outport  Port=3
  pol3_out : Outport  Port=4
  pol4_out : Outport  Port=5
  wires:
  In4/1 -> complex_addsub1/2(b)
  In3/1 -> complex_addsub1/1(a)
  mirror_spectrum/5(dout3) -> pol4_out/1
  mirror_spectrum/4(dout2) -> pol3_out/1
  mirror_spectrum/3(dout1) -> pol2_out/1
  mirror_spectrum/2(dout0) -> pol1_out/1
  mirror_spectrum/1(sync_out) -> sync_out/1
  In2/1 -> complex_addsub2/2(b)
  In1/1 -> complex_addsub2/1(a)
  sync/1 -> sync_delay_fast/1
  sync_delay_fast/1 -> reorder2/1(sync), Delay1/1
  complex_addsub1/1(a+b) -> reorder2/4(din2), mirror_spectrum/6(din2)
  complex_addsub1/2(a-b) -> reorder2/5(din3), mirror_spectrum/8(din3)
  reorder2/4(dout3) -> mirror_spectrum/9(reo_in3)
  reorder2/3(dout2) -> mirror_spectrum/7(reo_in2)
  reorder2/2(dout1) -> mirror_spectrum/5(reo_in1)
  reorder2/1(dout0) -> mirror_spectrum/3(reo_in0)
  Delay1/1 -> mirror_spectrum/1(sync)
  complex_addsub2/1(a+b) -> mirror_spectrum/2(din0), reorder2/2(din0)
  complex_addsub2/2(a-b) -> mirror_spectrum/4(din1), reorder2/3(din1)

== system monroe_library/FFT_Biplex_4x/biplex_4x_unscr ==
  even : Inport
  odd : Inport  Port=2
  sync : Inport  Port=3
  Constant1 : xbsIndex_r4/Constant  arith_type=Unsigned  const=511  n_bits=10  bin_pt=0  explicit_period=on  period=1  equ=P=C  opselect=C  inp2=PCIN>>17  opr=+  inp1=P  carry=CIN  dbl_ovrd=off  block_type=constant
  Constant2 : xbsIndex_r4/Constant  arith_type=Unsigned  const=1023  n_bits=10  bin_pt=0  explicit_period=on  period=1  equ=P=C  opselect=C  inp2=PCIN>>17  opr=+  inp1=P  carry=CIN  dbl_ovrd=off  block_type=constant
  Counter : xbsIndex_r4/Counter  cnt_type=Free Running  cnt_to=Inf  operation=Up  start_count=0  cnt_by_val=1  arith_type=Unsigned  n_bits=10  bin_pt=0  load_pin=off  rst=on  en=off  explicit_period=off  period=1  dbl_ovrd=off  use_behavioral_HDL=off  implementation=Fabric  use_rpm=on  block_type=counter
  Delay : xbsIndex_r4/Delay  en=off  latency=1  dbl_ovrd=off  reg_retiming=off  block_type=delay
  Mux{,1..3} (4 alike) : xbsIndex_r4/Mux  inputs=2  en=off  latency=1  precision=Full  arith_type="Signed  (2's comp)"  n_bits=8  bin_pt=2  quantization=Truncate  overflow=Wrap  dbl_ovrd=off  block_type=mux
  Relational : xbsIndex_r4/Relational  mode=a=b  en=off  latency=1  dbl_ovrd=off  block_type=relational
  Relational1 : xbsIndex_r4/Relational  mode=a=b  en=off  latency=1  dbl_ovrd=off  block_type=relational
  double_delay_bram_fast : monroe_library/double_delay_bram_fast  SystemSampleTime=-1  delay_len=512  bram_latency=2  register_counter=0
  dual_bit_reverse : Subsystem
  unscr_tail : monroe_library/unscr_tail  SystemSampleTime=-1  FFTSize=10  input_bit_width=18  bram_latency=2  reorder_din_latency=0
  pol1_out : Outport
  pol2_out : Outport  Port=2
  pol3_out : Outport  Port=3
  pol4_out : Outport  Port=4
  sync_out : Outport  Port=5
  wires:
  Delay/1 -> Mux3/3, Mux2/2, Mux1/3, Mux/2
  Counter/1 -> Relational1/2, Relational/1
  Relational/1 -> Mux3/1, Mux/1
  Relational1/1 -> Mux2/1, Mux1/1
  dual_bit_reverse/1(sync_out) -> unscr_tail/1, Counter/1
  dual_bit_reverse/2(dout0) -> Mux3/2, Mux2/3, Mux1/2, Mux/3
  unscr_tail/5 -> pol4_out/1
  unscr_tail/4 -> pol3_out/1
  unscr_tail/3 -> pol2_out/1
  unscr_tail/2 -> pol1_out/1
  unscr_tail/1 -> sync_out/1
  Mux2/1 -> unscr_tail/5
  Mux3/1 -> unscr_tail/4
  double_delay_bram_fast/2 -> unscr_tail/3
  double_delay_bram_fast/1 -> unscr_tail/2
  dual_bit_reverse/3(dout1) -> Delay/1
  odd/1 -> dual_bit_reverse/3(din1)
  even/1 -> dual_bit_reverse/2(din0)
  sync/1 -> dual_bit_reverse/1(sync)
  Mux/1 -> double_delay_bram_fast/2  "xlsub2_Mux_out1"
  Mux1/1 -> double_delay_bram_fast/1
  Constant1/1 -> Relational1/1
  Constant2/1 -> Relational/2
